simulink model "tarefa7e8"  (R2022b)
settings: Solver=VariableStepAuto  StartTime=0.0  StopTime=30  RelTol=1e-3
values from neighbouring files (symbols this model uses):
  d = -0.15    [lab7e8.m]
  R = 1.25    [lab7e8.m]
  T08 = 0.201    [lab7e8.m]
  td = 15    [lab7e8.m]
undefined symbols (not defined in the file or in its folder): Gden, Gnum, Gzden, Gznum
settings Model: Creator=hugo_  LastModifiedBy=hugo_

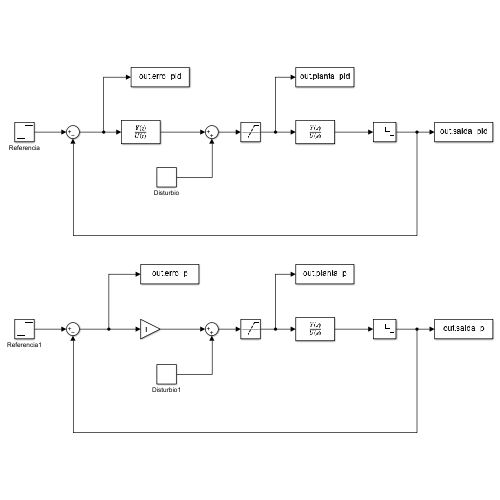
[thumbnail: Simulink's stored preview of the top-level diagram]
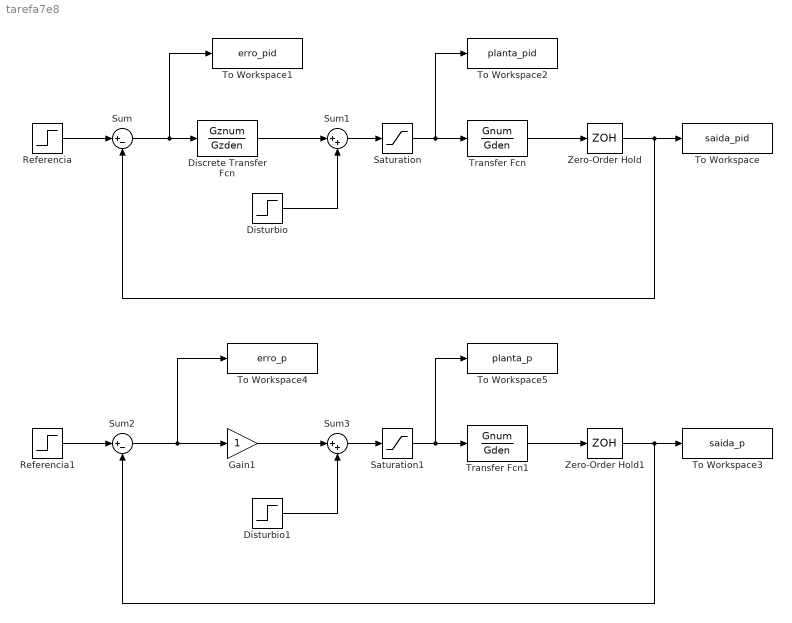
== system tarefa7e8 ==
  Discrete Transfer Fcn : DiscreteTransferFcn  Numerator=Gznum  Denominator=Gzden  SampleTime=T08
  Disturbio : Step  Time=td  After=d  SampleTime=0
  Disturbio1 : Step  Time=td  After=d  SampleTime=0
  Gain1 : Gain
  Referencia : Step  Time=0  After=R  SampleTime=0
  Referencia1 : Step  Time=0  After=R  SampleTime=0
  Saturation : Saturate  UpperLimit=10  LowerLimit=-10
  Saturation1 : Saturate  UpperLimit=10  LowerLimit=-10
  Sum : Sum  Inputs=|+-
  Sum1 : Sum  Inputs=|++
  Sum2 : Sum  Inputs=|+-
  Sum3 : Sum  Inputs=|++
  To Workspace : ToWorkspace  VariableName=saida_pid  SaveFormat=Timeseries  SampleTime=-1
  To Workspace1 : ToWorkspace  VariableName=erro_pid  SaveFormat=Timeseries  SampleTime=-1
  To Workspace2 : ToWorkspace  VariableName=planta_pid  SaveFormat=Timeseries  SampleTime=-1
  To Workspace3 : ToWorkspace  VariableName=saida_p  SaveFormat=Timeseries  SampleTime=-1
  To Workspace4 : ToWorkspace  VariableName=erro_p  SaveFormat=Timeseries  SampleTime=-1
  To Workspace5 : ToWorkspace  VariableName=planta_p  SaveFormat=Timeseries  SampleTime=-1
  Transfer Fcn : TransferFcn  Numerator=Gnum  Denominator=Gden
  Transfer Fcn1 : TransferFcn  Numerator=Gnum  Denominator=Gden
  Zero-Order Hold : ZeroOrderHold  SampleTime=T08
  Zero-Order Hold1 : ZeroOrderHold  SampleTime=T08
  wires:
  Sum/1 -> Discrete Transfer Fcn/1, To Workspace1/1
  Saturation/1 -> To Workspace2/1, Transfer Fcn/1
  Transfer Fcn/1 -> Zero-Order Hold/1
  Referencia/1 -> Sum/1
  Zero-Order Hold/1 -> Sum/2, To Workspace/1
  Sum1/1 -> Saturation/1
  Disturbio/1 -> Sum1/2
  Sum3/1 -> Saturation1/1
  Gain1/1 -> Sum3/1
  Saturation1/1 -> To Workspace5/1, Transfer Fcn1/1
  Sum2/1 -> To Workspace4/1, Gain1/1
  Transfer Fcn1/1 -> Zero-Order Hold1/1
  Zero-Order Hold1/1 -> Sum2/2, To Workspace3/1
  Disturbio1/1 -> Sum3/2
  Referencia1/1 -> Sum2/1
  Discrete Transfer Fcn/1 -> Sum1/1
